simulink model "GCI_Ctrl_PLL_C2000"  (R2024a)
settings: Solver=FixedStepDiscrete  StartTime=0.0  StopTime=8  FixedStep=Sim.ContSampleTime  RelTol=1e-3  EnableMultiTasking=on
values from neighbouring files (symbols this model uses):
  ADPTV = 1.3912    [ModelDD.sldd]
  Ctrl = 0    [ModelDD.sldd]
  EnableMonitors = 0    [ModelDD.sldd]
  FrcPwr = 1    [ModelDD.sldd]
  IdSp = 0.0    [ModelDD.sldd]
  IqSp = 0.0    [ModelDD.sldd]
  ModReq = 1    [ModelDD.sldd]
  PorISel = 0    [ModelDD.sldd]
  PSp = 0.0    [ModelDD.sldd]
  QSp = 0.0    [ModelDD.sldd]
  Sim : value not decoded    [ModelDD.sldd]
  Test = 0    [ModelDD.sldd]
  Var = 650.0    [ModelDD.sldd]
undefined symbols (not defined in the file or in its folder): DiscIntNeverNeededParam, Down, GPTRIP1SEL, GPTRIP2SEL, magnitude, P, TZ1, TZ2, Up
libraries: simulink x38, c2837xDlib x22, c2802xlib x15, slpidlib x9, spsMeanLib x9, spsCurrentMeasurementLib x7, spsThreePhaseVIMeasurementLib x5, spsVoltageMeasurementLib x5, spsTHDLib x4, spsSeriesRLCBranchLib x4, svdutilitieslib x3, c280xlib x3
(part 5 of 11)

== system GCI_Ctrl_PLL_C2000/C2000_SW/CtrlLoop/PWMs/HW ==
  Duty : Inport  OutDataTypeStr=single
  SPO : Inport  Port=2
  Bias3 : Bias  Bias=-100  SaturateOnIntegerOverflow=off
  Constant : Constant  Value=single([0 0 0])
  Constant2 : Constant  Value=single(zeros(1,6))
  Demux : Demux  Outputs=3
  Gain3 : Gain  Gain=-1  ParamDataTypeStr=single
  Mux : Mux  Inputs=2
  Switch : Switch  Criteria=u2 > Threshold  SaturateOnIntegerOverflow=off  InputSameDT=off
  Switch1 : Switch  Criteria=u2 > Threshold  SaturateOnIntegerOverflow=off  InputSameDT=off
  ePWM4 : c2802xlib/ePWM  PwmType=C2000_Type4  useModule=ePWM4  ePWMxLINKTBPRD=Not Linked  periodUnits=Seconds  timerSource=Specify via dialog  timerPeriod_clk=64000  timerPeriod_sec=1/(2*Var.PWM_Freq)  tbshadow=Counter equals to zero  countingMode=Up-Down  phaseActiveEnable=Disable  phaseDirection=Count down after sync  phaseActive=0  synchronizationEnable=off  dcaevt1Sync=off  dcbevt1Sync=off  synchronizationOption=Counter equals to zero (CTR=Zero)  dcbevt1SyncOut=off  dcaevt1SyncOut=off  cmpdSyncOut=off  cmpcSyncOut=off  cmpbSyncOut=off  zeroSyncOut=on  swfSyncOut=off  perSynchronizationOption=Counter equals to period (CTR=PRD)  clockPrescale=1  HSclockPrescale=1  enswap=off  ePWMxAStatus=on  ePWMxAactionLogic1=Do nothing  ePWMxAactionLogic2=Do nothing  ePWMxAactionLogic3=Clear  ePWMxAactionLogic4=Set  ePWMxAactionLogic5=Do nothing  ePWMxAactionLogic6=Do nothing  ePWMxACSFenable=off  ePWMxACSFvalue=Forcing disable  ePWMxASFreload=Zero  ePWMxBStatus=on  ePWMxBactionLogic1=Do nothing  ePWMxBactionLogic2=Do nothing  ePWMxBactionLogic3=Set  ePWMxBactionLogic4=Clear  ePWMxBactionLogic5=Do nothing  ePWMxBactionLogic6=Do nothing  ePWMxBCSFenable=off  ePWMxBCSFvalue=Forcing disable  ePWMxBSFreload=Zero  ePWNxBOutWay=off  ePWMxLINKCMPA=Not Linked  CMPAUnits=Percentages  CMPASource=Input port  CMPAValue_per=0  CMPAValue_clk=32000  enCMPAshadow=Counter equals to period (CTR=PRD)  ePWMxLINKCMPB=Not Linked  CMPBUnits=Percentages  CMPBSource=Specify via dialog  CMPBValue_per=100  CMPBValue_clk=32000  enCMPBshadow=Counter equals to period (CTR=PRD)  ePWMxLINKCMPC=Not Linked  CMPCUnits=Clock cycles  CMPCSource=Specify via dialog  CMPCValue_per=50  CMPCValue_clk=32000  enCMPCshadow=Counter equals to zero (CTR=Zero)  ePWMxLINKCMPD=Not Linked  CMPDUnits=Clock cycles  CMPDSource=Specify via dialog  CMPDValue_per=50  CMPDValue_clk=32000  enCMPDshadow=Counter equals to zero (CTR=Zero)  enableDBePWMxA=on  enableDBePWMxB=on  enhalfcycle=off  DBpolarity=Active high complementary (AHC)  DBedgeDelay=Positive  DBSource_ePWMxA=ePWMxA  DBSource_ePWMxB=ePWMxA  DBPeriodUnits=Clock cycles  DBperiodSource=Specify via dialog  REDperiod=Var.PWM_Deadtime*1e8  FEDperiod=Var.PWM_Deadtime*1e8  REDperiod_sec=0  FEDperiod_sec=0  LoadModeDBRED=Immediate without using shadow  LoadModeDBFED=Immediate without using shadow  adcstartModuleA=on  adcrequestEventA=First event  adcstartEventA=Digital Compare Module A Event 1 start of conversion (DCAEVT1.soc)  adcstartEventA_type2=Counter equals to period (CTR=PRD)  adcstartModuleB=off  adcrequestEventB=First event  adcstartEventB=Counter equals to zero (CTR=Zero)  adcstartEventB_type2=Counter equals to period (CTR=PRD)  intEn=on  intPrd=First event  intSel=Counter equals to zero (CTR=Zero)  intSel_type2=Counter equals to period (CTR=PRD)  hrpe=off  enHRPWM=off  HRPWM_LoadMode=Counter equals to either zero or period (CTR=ZERO or CTR=PRD)  HRPWM_CTLMode=Duty or Period control mode  HRPWM_EDGMode=Both edge  hrpeb=off  enHRPWMB=off  HRPWM_LoadModeB=Counter equals to zero (CTR=ZERO)  HRPWM_CTLModeB=Duty or Period control mode  HRPWM_EDGModeB=Both edge  enHRDBRED=off  enHRDBFED=off  enSFO=on  enautoconv=on  chopperEnable=off  chopperFrequency=1  chopperFirstwidth=1  chopperDuty=12.5%  tripZonesource=Specify via dialog  tzselOSHT1=off  tzselOSHT2=off  tzselOSHT3=off  tzselOSHT4=off  tzselOSHT5=off  tzselOSHT6=off  tzselOSHDCAEV1=off  tzselOSHDCBEV1=off  tzselCBC1=on  tzselCBC2=off  tzselCBC3=off  tzselCBC4=off  tzselCBC5=off  tzselCBC6=off  tzselCBCDCAEV2=off  tzselCBCDCBEV2=off  enTzOstIntr=off  enTzCbcIntr=off  enTzDCAEVT1Intr=off  enTzDCAEVT2Intr=off  enTzDCBEVT1Intr=off  enTzDCBEVT2Intr=off  tzclrCBCLatch=Counter equals to zero (CTR=Zero)  ePWMxAforced=Low  ePWMxBforced=Low  DCAEVT1forced=No action  DCBEVT1forced=No action  DCAEVT2forced=No action  DCBEVT2forced=No action  dcah=Trip Zone 1 input (TZ1)  dcal=Trip Zone 2 input (TZ2)  dcbh=Trip Zone 1 input (TZ1)  dcbl=Trip Zone 2 input (TZ2)  dcah_type2=GPTRIP1SEL/(TZ1)  dcal_type2=GPTRIP2SEL/(TZ2)  dcbh_type2=GPTRIP1SEL/(TZ1)  dcbl_type2=GPTRIP2SEL/(TZ2)  gendcaevt1=Event disabled  gendcaevt2=Event disabled  gendcbevt1=Event disabled  gendcbevt2=Event disabled  dcaevt1src=DCAEVT1 with sync  dcaevt2src=DCAEVT2 with sync  dcbevt1src=DCBEVT1 with sync  dcbevt2src=DCBEVT2 with sync  pulsesel=Counter equals to zero (CTR=Zero)  blankinv=off  blankoffset=0  blankwidth=0  evsrcsel=Filtered version of DCAEVT1 (DCAEVT1FILT)  encape=off
  ePWM5 : c2802xlib/ePWM  PwmType=C2000_Type4  useModule=ePWM5  ePWMxLINKTBPRD=Not Linked  periodUnits=Seconds  timerSource=Specify via dialog  timerPeriod_clk=64000  timerPeriod_sec=1/(2*Var.PWM_Freq)  tbshadow=Counter equals to zero  countingMode=Up-Down  phaseActiveEnable=Set counter to phase value specified via dialog  phaseDirection=Count up after sync  phaseActive=0  synchronizationEnable=off  dcaevt1Sync=off  dcbevt1Sync=off  synchronizationOption=Pass through (EPWMxSYNCI or SWFSYNC)  dcbevt1SyncOut=off  dcaevt1SyncOut=off  cmpdSyncOut=off  cmpcSyncOut=off  cmpbSyncOut=off  zeroSyncOut=off  swfSyncOut=on  perSynchronizationOption=Counter equals to period (CTR=PRD)  clockPrescale=1  HSclockPrescale=1  enswap=off  ePWMxAStatus=on  ePWMxAactionLogic1=Do nothing  ePWMxAactionLogic2=Do nothing  ePWMxAactionLogic3=Clear  ePWMxAactionLogic4=Set  ePWMxAactionLogic5=Do nothing  ePWMxAactionLogic6=Do nothing  ePWMxACSFenable=off  ePWMxACSFvalue=Forcing disable  ePWMxASFreload=Zero  ePWMxBStatus=on  ePWMxBactionLogic1=Do nothing  ePWMxBactionLogic2=Do nothing  ePWMxBactionLogic3=Set  ePWMxBactionLogic4=Clear  ePWMxBactionLogic5=Do nothing  ePWMxBactionLogic6=Do nothing  ePWMxBCSFenable=off  ePWMxBCSFvalue=Forcing disable  ePWMxBSFreload=Zero  ePWNxBOutWay=off  ePWMxLINKCMPA=Not Linked  CMPAUnits=Percentages  CMPASource=Input port  CMPAValue_per=0  CMPAValue_clk=32000  enCMPAshadow=Counter equals to period (CTR=PRD)  ePWMxLINKCMPB=Not Linked  CMPBUnits=Percentages  CMPBSource=Specify via dialog  CMPBValue_per=100  CMPBValue_clk=32000  enCMPBshadow=Counter equals to period (CTR=PRD)  ePWMxLINKCMPC=Not Linked  CMPCUnits=Clock cycles  CMPCSource=Specify via dialog  CMPCValue_per=50  CMPCValue_clk=32000  enCMPCshadow=Counter equals to zero (CTR=Zero)  ePWMxLINKCMPD=Not Linked  CMPDUnits=Clock cycles  CMPDSource=Specify via dialog  CMPDValue_per=50  CMPDValue_clk=32000  enCMPDshadow=Counter equals to zero (CTR=Zero)  enableDBePWMxA=on  enableDBePWMxB=on  enhalfcycle=off  DBpolarity=Active high complementary (AHC)  DBedgeDelay=Positive  DBSource_ePWMxA=ePWMxA  DBSource_ePWMxB=ePWMxA  DBPeriodUnits=Clock cycles  DBperiodSource=Specify via dialog  REDperiod=Var.PWM_Deadtime*1e8  FEDperiod=Var.PWM_Deadtime*1e8  REDperiod_sec=0  FEDperiod_sec=0  LoadModeDBRED=Immediate without using shadow  LoadModeDBFED=Immediate without using shadow  adcstartModuleA=off  adcrequestEventA=First event  adcstartEventA=Digital Compare Module A Event 1 start of conversion (DCAEVT1.soc)  adcstartEventA_type2=Digital Compare Module A Event 1 start of conversion (DCAEVT1.soc)  adcstartModuleB=off  adcrequestEventB=First event  adcstartEventB=Counter equals to zero (CTR=Zero)  adcstartEventB_type2=Counter equals to zero (CTR=Zero)  intEn=off  intPrd=First event  intSel=Counter equals to zero (CTR=Zero)  intSel_type2=Counter equals to zero (CTR=Zero)  hrpe=off  enHRPWM=off  HRPWM_LoadMode=Counter equals to either zero or period (CTR=ZERO or CTR=PRD)  HRPWM_CTLMode=Duty or Period control mode  HRPWM_EDGMode=Both edge  hrpeb=off  enHRPWMB=off  HRPWM_LoadModeB=Counter equals to zero (CTR=ZERO)  HRPWM_CTLModeB=Duty or Period control mode  HRPWM_EDGModeB=Both edge  enHRDBRED=off  enHRDBFED=off  enSFO=on  enautoconv=on  chopperEnable=off  chopperFrequency=1  chopperFirstwidth=1  chopperDuty=12.5%  tripZonesource=Specify via dialog  tzselOSHT1=off  tzselOSHT2=off  tzselOSHT3=off  tzselOSHT4=off  tzselOSHT5=off  tzselOSHT6=off  tzselOSHDCAEV1=off  tzselOSHDCBEV1=off  tzselCBC1=on  tzselCBC2=off  tzselCBC3=off  tzselCBC4=off  tzselCBC5=off  tzselCBC6=off  tzselCBCDCAEV2=off  tzselCBCDCBEV2=off  enTzOstIntr=off  enTzCbcIntr=off  enTzDCAEVT1Intr=off  enTzDCAEVT2Intr=off  enTzDCBEVT1Intr=off  enTzDCBEVT2Intr=off  tzclrCBCLatch=Counter equals to zero (CTR=Zero)  ePWMxAforced=Low  ePWMxBforced=Low  DCAEVT1forced=No action  DCBEVT1forced=No action  DCAEVT2forced=No action  DCBEVT2forced=No action  dcah=Trip Zone 1 input (TZ1)  dcal=Trip Zone 2 input (TZ2)  dcbh=Trip Zone 1 input (TZ1)  dcbl=Trip Zone 2 input (TZ2)  dcah_type2=GPTRIP1SEL/(TZ1)  dcal_type2=GPTRIP2SEL/(TZ2)  dcbh_type2=GPTRIP1SEL/(TZ1)  dcbl_type2=GPTRIP2SEL/(TZ2)  gendcaevt1=Event disabled  gendcaevt2=Event disabled  gendcbevt1=Event disabled  gendcbevt2=Event disabled  dcaevt1src=DCAEVT1 with sync  dcaevt2src=DCAEVT2 with sync  dcbevt1src=DCBEVT1 with sync  dcbevt2src=DCBEVT2 with sync  pulsesel=Counter equals to zero (CTR=Zero)  blankinv=off  blankoffset=0  blankwidth=0  evsrcsel=Filtered version of DCAEVT1 (DCAEVT1FILT)  encape=off
  ePWM6 : c2802xlib/ePWM  PwmType=C2000_Type4  useModule=ePWM6  ePWMxLINKTBPRD=Not Linked  periodUnits=Seconds  timerSource=Specify via dialog  timerPeriod_clk=64000  timerPeriod_sec=1/(2*Var.PWM_Freq)  tbshadow=Counter equals to zero  countingMode=Up-Down  phaseActiveEnable=Set counter to phase value specified via dialog  phaseDirection=Count up after sync  phaseActive=0  synchronizationEnable=off  dcaevt1Sync=off  dcbevt1Sync=off  synchronizationOption=Disable  dcbevt1SyncOut=off  dcaevt1SyncOut=off  cmpdSyncOut=off  cmpcSyncOut=off  cmpbSyncOut=off  zeroSyncOut=off  swfSyncOut=off  perSynchronizationOption=Counter equals to period (CTR=PRD)  clockPrescale=1  HSclockPrescale=1  enswap=off  ePWMxAStatus=on  ePWMxAactionLogic1=Do nothing  ePWMxAactionLogic2=Do nothing  ePWMxAactionLogic3=Clear  ePWMxAactionLogic4=Set  ePWMxAactionLogic5=Do nothing  ePWMxAactionLogic6=Do nothing  ePWMxACSFenable=off  ePWMxACSFvalue=Forcing disable  ePWMxASFreload=Zero  ePWMxBStatus=on  ePWMxBactionLogic1=Do nothing  ePWMxBactionLogic2=Do nothing  ePWMxBactionLogic3=Set  ePWMxBactionLogic4=Clear  ePWMxBactionLogic5=Do nothing  ePWMxBactionLogic6=Do nothing  ePWMxBCSFenable=off  ePWMxBCSFvalue=Forcing disable  ePWMxBSFreload=Zero  ePWNxBOutWay=off  ePWMxLINKCMPA=Not Linked  CMPAUnits=Percentages  CMPASource=Input port  CMPAValue_per=0  CMPAValue_clk=32000  enCMPAshadow=Counter equals to period (CTR=PRD)  ePWMxLINKCMPB=Not Linked  CMPBUnits=Percentages  CMPBSource=Specify via dialog  CMPBValue_per=100  CMPBValue_clk=32000  enCMPBshadow=Counter equals to period (CTR=PRD)  ePWMxLINKCMPC=Not Linked  CMPCUnits=Clock cycles  CMPCSource=Specify via dialog  CMPCValue_per=50  CMPCValue_clk=32000  enCMPCshadow=Counter equals to zero (CTR=Zero)  ePWMxLINKCMPD=Not Linked  CMPDUnits=Clock cycles  CMPDSource=Specify via dialog  CMPDValue_per=50  CMPDValue_clk=32000  enCMPDshadow=Counter equals to zero (CTR=Zero)  enableDBePWMxA=on  enableDBePWMxB=on  enhalfcycle=off  DBpolarity=Active high complementary (AHC)  DBedgeDelay=Positive  DBSource_ePWMxA=ePWMxA  DBSource_ePWMxB=ePWMxA  DBPeriodUnits=Clock cycles  DBperiodSource=Specify via dialog  REDperiod=Var.PWM_Deadtime*1e8  FEDperiod=Var.PWM_Deadtime*1e8  REDperiod_sec=0  FEDperiod_sec=0  LoadModeDBRED=Immediate without using shadow  LoadModeDBFED=Immediate without using shadow  adcstartModuleA=off  adcrequestEventA=First event  adcstartEventA=Digital Compare Module A Event 1 start of conversion (DCAEVT1.soc)  adcstartEventA_type2=Digital Compare Module A Event 1 start of conversion (DCAEVT1.soc)  adcstartModuleB=off  adcrequestEventB=First event  adcstartEventB=Counter equals to zero (CTR=Zero)  adcstartEventB_type2=Counter equals to zero (CTR=Zero)  intEn=off  intPrd=First event  intSel=Counter equals to zero (CTR=Zero)  intSel_type2=Counter equals to zero (CTR=Zero)  hrpe=off  enHRPWM=off  HRPWM_LoadMode=Counter equals to either zero or period (CTR=ZERO or CTR=PRD)  HRPWM_CTLMode=Duty or Period control mode  HRPWM_EDGMode=Both edge  hrpeb=off  enHRPWMB=off  HRPWM_LoadModeB=Counter equals to zero (CTR=ZERO)  HRPWM_CTLModeB=Duty or Period control mode  HRPWM_EDGModeB=Both edge  enHRDBRED=off  enHRDBFED=off  enSFO=on  enautoconv=on  chopperEnable=off  chopperFrequency=1  chopperFirstwidth=1  chopperDuty=12.5%  tripZonesource=Specify via dialog  tzselOSHT1=off  tzselOSHT2=off  tzselOSHT3=off  tzselOSHT4=off  tzselOSHT5=off  tzselOSHT6=off  tzselOSHDCAEV1=off  tzselOSHDCBEV1=off  tzselCBC1=on  tzselCBC2=off  tzselCBC3=off  tzselCBC4=off  tzselCBC5=off  tzselCBC6=off  tzselCBCDCAEV2=off  tzselCBCDCBEV2=off  enTzOstIntr=off  enTzCbcIntr=off  enTzDCAEVT1Intr=off  enTzDCAEVT2Intr=off  enTzDCBEVT1Intr=off  enTzDCBEVT2Intr=off  tzclrCBCLatch=Counter equals to zero (CTR=Zero)  ePWMxAforced=Low  ePWMxBforced=Low  DCAEVT1forced=No action  DCBEVT1forced=No action  DCAEVT2forced=No action  DCBEVT2forced=No action  dcah=Trip Zone 1 input (TZ1)  dcal=Trip Zone 2 input (TZ2)  dcbh=Trip Zone 1 input (TZ1)  dcbl=Trip Zone 2 input (TZ2)  dcah_type2=GPTRIP1SEL/(TZ1)  dcal_type2=GPTRIP2SEL/(TZ2)  dcbh_type2=GPTRIP1SEL/(TZ1)  dcbl_type2=GPTRIP2SEL/(TZ2)  gendcaevt1=Event disabled  gendcaevt2=Event disabled  gendcbevt1=Event disabled  gendcbevt2=Event disabled  dcaevt1src=DCAEVT1 with sync  dcaevt2src=DCAEVT2 with sync  dcbevt1src=DCBEVT1 with sync  dcbevt2src=DCBEVT2 with sync  pulsesel=Counter equals to zero (CTR=Zero)  blankinv=off  blankoffset=0  blankwidth=0  evsrcsel=Filtered version of DCAEVT1 (DCAEVT1FILT)  encape=off
  DutyOut : Outport  VectorParamsAs1DForOutWhenUnconnected=off
  wires:
  Switch/1 -> Demux/1, Mux/1, Bias3/1
  Demux/1 -> ePWM4/1
  Switch1/1 -> DutyOut/1
  Demux/3 -> ePWM6/1
  Duty/1 -> Switch/3
  Constant/1 -> Switch/1
  Demux/2 -> ePWM5/1
  Constant2/1 -> Switch1/1
  SPO/1 -> [A1]
  [A1] -> Switch1/2
  [A1] -> Switch/2
  Bias3/1 -> Gain3/1
  Gain3/1 -> Mux/2
  Mux/1 -> Switch1/3

== system GCI_Ctrl_PLL_C2000/C2000_SW/CtrlLoop/PWMs/SIM ==
  Duty : Inport  OutDataTypeStr=single
  SPO : Inport  Port=2
  Bias2 : Bias  Bias=-100  SaturateOnIntegerOverflow=off
  Constant : Constant  OutDataTypeStr=boolean
  Constant1 : Constant  Value=single([0 0 0 0 0 0])
  Gain1 : Gain  Gain=-1  ParamDataTypeStr=single
  Manual Switch : ManualSwitch  CurrentSetting=0
  Mux : Mux  Inputs=2
  Switch : Switch  Criteria=u2 > Threshold  SaturateOnIntegerOverflow=off  InputSameDT=off
  DutyOut : Outport  VectorParamsAs1DForOutWhenUnconnected=off
  wires:
  Manual Switch/1 -> Switch/2
  Duty/1 -> Mux/1, Bias2/1
  Constant/1 -> Manual Switch/1
  Constant1/1 -> Switch/1
  Switch/1 -> DutyOut/1  "DutyOut"
  Mux/1 -> Switch/3
  SPO/1 -> Manual Switch/2
  Bias2/1 -> Gain1/1
  Gain1/1 -> Mux/2

== system GCI_Ctrl_PLL_C2000/C2000_SW/CtrlLoop/RMS/LPF2 ==
  u : Inport
  Alpha : Gain  Gain=(2-w*Ts)/(2+w*Ts)
  Beta : Gain  Gain=(w*Ts)/(2+w*Ts)
  Delay1 : Delay  DelayLength=1  InitialCondition=y_0
  Delay2 : Delay  DelayLength=1
  Sum1 : Sum  Inputs=++|
  Sum2 : Sum  Inputs=|++
  y : Outport  VectorParamsAs1DForOutWhenUnconnected=off
  wires:
  Sum2/1 -> y/1, Delay1/1
  Beta/1 -> Sum2/1
  Sum1/1 -> Beta/1
  Delay2/1 -> Sum1/2
  Alpha/1 -> Sum2/2
  Delay1/1 -> Alpha/1  "y(n-1)"
  u/1 -> Delay2/1, Sum1/1

== system GCI_Ctrl_PLL_C2000/C2000_SW/CtrlLoop/RMS1/LPF2 ==
  u : Inport
  Alpha : Gain  Gain=(2-w*Ts)/(2+w*Ts)
  Beta : Gain  Gain=(w*Ts)/(2+w*Ts)
  Delay1 : Delay  DelayLength=1  InitialCondition=y_0
  Delay2 : Delay  DelayLength=1
  Sum1 : Sum  Inputs=++|
  Sum2 : Sum  Inputs=|++
  y : Outport  VectorParamsAs1DForOutWhenUnconnected=off
  wires:
  u/1 -> Sum1/1, Delay2/1
  Delay1/1 -> Alpha/1  "y(n-1)"
  Alpha/1 -> Sum2/2
  Delay2/1 -> Sum1/2
  Sum1/1 -> Beta/1
  Beta/1 -> Sum2/1
  Sum2/1 -> Delay1/1, y/1

== system GCI_Ctrl_PLL_C2000/C2000_SW/MnrErr/Monitoring/ADC_OORH ==
  u : Inport
  Bias : Bias  Bias=single(-0.5)  SaturateOnIntegerOverflow=off
  Compare To Constant : simulink/Logic and Bit Operations/Compare To Constant  relop=>=  const=Lim  OutDataTypeStr=uint8
  Compare To Constant1 : simulink/Logic and Bit Operations/Compare To Constant  relop===  const=single(2)  OutDataTypeStr=boolean
  Compare To Constant2 : simulink/Logic and Bit Operations/Compare To Constant  relop===  const=single(-1.5)  OutDataTypeStr=boolean
  Compare To Constant3 : simulink/Logic and Bit Operations/Compare To Constant  relop=<=  const=LimN  OutDataTypeStr=uint8
  Constant : Constant  Value=single(0)
  Constant1 : Constant  Value=UorL
  Discrete-Time Integrator2 : DiscreteIntegrator  gainval=single(1/Tmon)  SampleTime=-1  OutDataTypeStr=single  LimitOutput=on  UpperSaturationLimit=single(1)  LowerSaturationLimit=single(0)  ShowSaturationPort=on  ICPrevOutput=DiscIntNeverNeededParam  ICPrevScaledInput=DiscIntNeverNeededParam
  Gain : Gain  Gain=single(1.5)  ParamDataTypeStr=single
  OR : Logic  Operator=OR  IconShape=distinctive  AllPortsSameDT=off  OutDataTypeStr=boolean
  Relay : Relay  OnSwitchValue=1  OffSwitchValue=0
  Sum : Sum  Inputs=|++
  Switch : Switch  Threshold=1  SaturateOnIntegerOverflow=off  InputSameDT=off
  Switch1 : Switch  Threshold=1  SaturateOnIntegerOverflow=off  InputSameDT=off
  Unit Delay : UnitDelay  SampleTime=-1  HasFrameUpgradeWarning=on
  err : Outport
  wires:
  Unit Delay/1 -> Sum/1
  Discrete-Time Integrator2/1 -> Relay/1
  Constant/1 -> Switch/1
  Switch/1 -> Discrete-Time Integrator2/1
  Discrete-Time Integrator2/2 -> Unit Delay/1
  Relay/1 -> err/1
  Sum/1 -> Compare To Constant2/1, Compare To Constant1/1
  Compare To Constant2/1 -> OR/1
  Compare To Constant1/1 -> OR/2
  OR/1 -> Switch/2
  Switch1/1 -> Gain/1
  Gain/1 -> Bias/1
  Bias/1 -> Switch/3, Sum/2
  Compare To Constant3/1 -> Switch1/3
  Compare To Constant/1 -> Switch1/1
  Constant1/1 -> Switch1/2
  u/1 -> Compare To Constant/1, Compare To Constant3/1

== system GCI_Ctrl_PLL_C2000/C2000_SW/MnrErr/Monitoring/ADC_OORL ==
  u : Inport
  Bias : Bias  Bias=single(-0.5)  SaturateOnIntegerOverflow=off
  Compare To Constant : simulink/Logic and Bit Operations/Compare To Constant  relop=>=  const=Lim  OutDataTypeStr=uint8
  Compare To Constant1 : simulink/Logic and Bit Operations/Compare To Constant  relop===  const=single(2)  OutDataTypeStr=boolean
  Compare To Constant2 : simulink/Logic and Bit Operations/Compare To Constant  relop===  const=single(-1.5)  OutDataTypeStr=boolean
  Compare To Constant3 : simulink/Logic and Bit Operations/Compare To Constant  relop=<=  const=LimN  OutDataTypeStr=uint8
  Constant : Constant  Value=single(0)
  Constant1 : Constant  Value=UorL
  Discrete-Time Integrator2 : DiscreteIntegrator  gainval=single(1/Tmon)  SampleTime=-1  OutDataTypeStr=single  LimitOutput=on  UpperSaturationLimit=single(1)  LowerSaturationLimit=single(0)  ShowSaturationPort=on  ICPrevOutput=DiscIntNeverNeededParam  ICPrevScaledInput=DiscIntNeverNeededParam
  Gain : Gain  Gain=single(1.5)  ParamDataTypeStr=single
  OR : Logic  Operator=OR  IconShape=distinctive  AllPortsSameDT=off  OutDataTypeStr=boolean
  Relay : Relay  OnSwitchValue=1  OffSwitchValue=0
  Sum : Sum  Inputs=|++
  Switch : Switch  Threshold=1  SaturateOnIntegerOverflow=off  InputSameDT=off
  Switch1 : Switch  Threshold=1  SaturateOnIntegerOverflow=off  InputSameDT=off
  Unit Delay : UnitDelay  SampleTime=-1  HasFrameUpgradeWarning=on
  err : Outport
  wires:
  u/1 -> Compare To Constant3/1, Compare To Constant/1
  Constant1/1 -> Switch1/2
  Compare To Constant/1 -> Switch1/1
  Compare To Constant3/1 -> Switch1/3
  Bias/1 -> Sum/2, Switch/3
  Gain/1 -> Bias/1
  Switch1/1 -> Gain/1
  OR/1 -> Switch/2
  Compare To Constant1/1 -> OR/2
  Compare To Constant2/1 -> OR/1
  Sum/1 -> Compare To Constant1/1, Compare To Constant2/1
  Relay/1 -> err/1
  Discrete-Time Integrator2/2 -> Unit Delay/1
  Switch/1 -> Discrete-Time Integrator2/1
  Constant/1 -> Switch/1
  Discrete-Time Integrator2/1 -> Relay/1
  Unit Delay/1 -> Sum/1

== system GCI_Ctrl_PLL_C2000/C2000_SW/MnrErr/Monitoring/HvdcUOV ==
  u : Inport
  Bias : Bias  Bias=single(-0.01)  SaturateOnIntegerOverflow=off
  Compare To Constant : simulink/Logic and Bit Operations/Compare To Constant  relop=>=  const=Lim  OutDataTypeStr=uint8
  Compare To Constant1 : simulink/Logic and Bit Operations/Compare To Constant  relop===  const=single(2)  OutDataTypeStr=boolean
  Compare To Constant2 : simulink/Logic and Bit Operations/Compare To Constant  relop===  const=single(-1.5)  OutDataTypeStr=boolean
  Compare To Constant3 : simulink/Logic and Bit Operations/Compare To Constant  relop=<=  const=LimN  OutDataTypeStr=uint8
  Constant : Constant  Value=single(0)
  Constant1 : Constant  Value=UorL
  Discrete-Time Integrator2 : DiscreteIntegrator  gainval=single(1/Tmon)  SampleTime=-1  OutDataTypeStr=single  LimitOutput=on  UpperSaturationLimit=single(1)  LowerSaturationLimit=single(0)  ShowSaturationPort=on  ICPrevOutput=DiscIntNeverNeededParam  ICPrevScaledInput=DiscIntNeverNeededParam
  Gain : Gain  Gain=single(1.01)  ParamDataTypeStr=single
  OR : Logic  Operator=OR  IconShape=distinctive  AllPortsSameDT=off  OutDataTypeStr=boolean
  Relay : Relay  OnSwitchValue=1  OffSwitchValue=0
  Sum : Sum  Inputs=|++
  Switch : Switch  Threshold=1  SaturateOnIntegerOverflow=off  InputSameDT=off
  Switch1 : Switch  Threshold=1  SaturateOnIntegerOverflow=off  InputSameDT=off
  Unit Delay : UnitDelay  SampleTime=-1  HasFrameUpgradeWarning=on
  err : Outport
  wires:
  u/1 -> Compare To Constant3/1, Compare To Constant/1
  Constant1/1 -> Switch1/2
  Compare To Constant/1 -> Switch1/1
  Compare To Constant3/1 -> Switch1/3
  Bias/1 -> Sum/2, Switch/3
  Gain/1 -> Bias/1
  Switch1/1 -> Gain/1
  OR/1 -> Switch/2
  Compare To Constant1/1 -> OR/2
  Compare To Constant2/1 -> OR/1
  Sum/1 -> Compare To Constant1/1, Compare To Constant2/1
  Relay/1 -> err/1
  Discrete-Time Integrator2/2 -> Unit Delay/1
  Switch/1 -> Discrete-Time Integrator2/1
  Constant/1 -> Switch/1
  Discrete-Time Integrator2/1 -> Relay/1
  Unit Delay/1 -> Sum/1

== system GCI_Ctrl_PLL_C2000/C2000_SW/MnrErr/Monitoring/RMS_OC ==
  u : Inport
  Bias : Bias  Bias=single(-0.01)  SaturateOnIntegerOverflow=off
  Compare To Constant : simulink/Logic and Bit Operations/Compare To Constant  relop=>=  const=Lim  OutDataTypeStr=uint8
  Compare To Constant1 : simulink/Logic and Bit Operations/Compare To Constant  relop===  const=single(2)  OutDataTypeStr=boolean
  Compare To Constant2 : simulink/Logic and Bit Operations/Compare To Constant  relop===  const=single(-1.5)  OutDataTypeStr=boolean
  Compare To Constant3 : simulink/Logic and Bit Operations/Compare To Constant  relop=<=  const=LimN  OutDataTypeStr=uint8
  Constant : Constant  Value=single(0)
  Constant1 : Constant  Value=UorL
  Discrete-Time Integrator2 : DiscreteIntegrator  gainval=single(1/Tmon)  SampleTime=-1  OutDataTypeStr=single  LimitOutput=on  UpperSaturationLimit=single(1)  LowerSaturationLimit=single(0)  ShowSaturationPort=on  ICPrevOutput=DiscIntNeverNeededParam  ICPrevScaledInput=DiscIntNeverNeededParam
  Gain : Gain  Gain=single(1.01)  ParamDataTypeStr=single
  OR : Logic  Operator=OR  IconShape=distinctive  AllPortsSameDT=off  OutDataTypeStr=boolean
  Relay : Relay  OnSwitchValue=1  OffSwitchValue=0
  Sum : Sum  Inputs=|++
  Switch : Switch  Threshold=1  SaturateOnIntegerOverflow=off  InputSameDT=off
  Switch1 : Switch  Threshold=1  SaturateOnIntegerOverflow=off  InputSameDT=off
  Unit Delay : UnitDelay  SampleTime=-1  HasFrameUpgradeWarning=on
  err : Outport
  wires:
  Unit Delay/1 -> Sum/1
  Discrete-Time Integrator2/1 -> Relay/1
  Constant/1 -> Switch/1
  Switch/1 -> Discrete-Time Integrator2/1
  Discrete-Time Integrator2/2 -> Unit Delay/1
  Relay/1 -> err/1
  Sum/1 -> Compare To Constant2/1, Compare To Constant1/1
  Compare To Constant2/1 -> OR/1
  Compare To Constant1/1 -> OR/2
  OR/1 -> Switch/2
  Switch1/1 -> Gain/1
  Gain/1 -> Bias/1
  Bias/1 -> Switch/3, Sum/2
  Compare To Constant3/1 -> Switch1/3
  Compare To Constant/1 -> Switch1/1
  Constant1/1 -> Switch1/2
  u/1 -> Compare To Constant/1, Compare To Constant3/1

== system GCI_Ctrl_PLL_C2000/PowerSystem/Actual System/PWMGen2/Deadtime ==
  In1 : Inport
  AND : Logic  IconShape=distinctive  AllPortsSameDT=off  OutDataTypeStr=boolean
  Data Type Conversion : DataTypeConversion  OutDataTypeStr=double  SaturateOnIntegerOverflow=off  RndMeth=Floor
  Data Type Conversion1 : DataTypeConversion  SaturateOnIntegerOverflow=off  RndMeth=Floor
  Transport Delay : TransportDelay  DelayTime=double(Var.PWM.Freq)
  Out1 : Outport  VectorParamsAs1DForOutWhenUnconnected=off
  wires:
  Transport Delay/1 -> AND/1
  In1/1 -> Data Type Conversion/1
  AND/1 -> Data Type Conversion1/1
  Data Type Conversion/1 -> Transport Delay/1, AND/2
  Data Type Conversion1/1 -> Out1/1

== system GCI_Ctrl_PLL_C2000/PowerSystem/Meas/Fault Injection/3PhaseToGnd ==
  Add7 : Sum
  Constant : Constant  Value=Mag
  Constant1 : Constant  Value=Frq*2*pi
  Constant2 : Constant  Value=Pha*pi/180
  Constant3 : Constant  Value=HarmOrd  VectorParams1D=off
  Constant4 : Constant  Value=IntHarmOrd  VectorParams1D=off
  Constant5 : Constant  Value=2*pi
  Cos1 : Trigonometry  Operator=cos
  Cos3 : Trigonometry  Operator=cos
  Cos8 : Trigonometry  Operator=cos
  Discrete-Time Integrator2 : DiscreteIntegrator  IntegratorMethod=Integration: Trapezoidal  SampleTime=-1  ICPrevOutput=DiscIntNeverNeededParam  ICPrevScaledInput=DiscIntNeverNeededParam
  Frq : Step  Time=FrqStpT  After=FrqStp*2*pi  SampleTime=0
  Gain : Gain  Gain=DcOff
  Harm : Step  Time=HarmStp  After=Harm  SampleTime=0  VectorParams1D=off
  Harm1 : Step  Time=IntHarmStp  After=IntHarm  SampleTime=0  VectorParams1D=off
  Mag : Step  Time=MagStpT  Before=1  After=MagStpPerc  SampleTime=0
  Matrix Multiply{,1..3} (4 alike) : Product  Multiplication=Matrix(*)
  Mod : Math  Operator=mod  SignedPower=on
  Phase : Step  Time=PhaStpT  After=(PhaStpPerc)*pi/180  SampleTime=0
  Product{,1,3,8} (4 alike) : Product
  Sum : Sum  Inputs=|++
  Sum of Elements : Sum  Inputs=+  CollapseMode=Specified dimension  CollapseDim=2
  Sum of Elements1 : Sum  Inputs=+  CollapseMode=Specified dimension  CollapseDim=2
  Sum of Elements2 : Sum  Inputs=+
  Sum1 : Sum  Inputs=|++
  Sum2 : Sum  Inputs=+--
  Sum3 : Sum  Inputs=++|
  Uact : Scope  NumInputPorts=2
  Wave : Outport  VectorParamsAs1DForOutWhenUnconnected=off
  wires:
  Sum of Elements2/1 -> Sum/2
  Mod/1 -> Uact/1  "wt_act"
  Constant5/1 -> Mod/2
  Gain/1 -> Sum3/1
  Sum3/1 -> Wave/1, Uact/2  "Uabc_act"
  Add7/1 -> Matrix Multiply/1, Matrix Multiply2/1, Cos3/1
  Product/1 -> Gain/1, Product3/2, Matrix Multiply1/1, Matrix Multiply3/1
  Matrix Multiply2/1 -> Cos1/1
  Matrix Multiply3/1 -> Product1/1
  Cos1/1 -> Product1/2
  Product1/1 -> Sum of Elements1/1
  Constant4/1 -> Matrix Multiply2/2
  Harm1/1 -> Matrix Multiply3/2
  Sum of Elements1/1 -> Sum2/3
  Sum2/1 -> Sum3/2
  Sum of Elements/1 -> Sum2/2
  Harm/1 -> Matrix Multiply1/2
  Constant3/1 -> Matrix Multiply/2
  Product8/1 -> Sum of Elements/1
  Cos8/1 -> Product8/2
  Matrix Multiply1/1 -> Product8/1
  Matrix Multiply/1 -> Cos8/1
  Constant2/1 -> Sum1/1
  Phase/1 -> Sum1/2
  Constant/1 -> Product/1
  Mag/1 -> Product/2
  Frq/1 -> Sum of Elements2/1
  Constant1/1 -> Sum/1
  Sum/1 -> Discrete-Time Integrator2/1
  Discrete-Time Integrator2/1 -> Add7/1, Mod/1  "wt_act"
  Product3/1 -> Sum2/1
  Sum1/1 -> Add7/2
  Cos3/1 -> Product3/1

== system GCI_Ctrl_PLL_C2000/PowerSystem/Meas/Fault Injection/FreqVar ==
  Add7 : Sum
  Constant : Constant  Value=Mag
  Constant1 : Constant  Value=Frq*2*pi
  Constant2 : Constant  Value=Pha*pi/180
  Constant3 : Constant  Value=HarmOrd  VectorParams1D=off
  Constant4 : Constant  Value=IntHarmOrd  VectorParams1D=off
  Constant5 : Constant  Value=2*pi
  Cos1 : Trigonometry  Operator=cos
  Cos3 : Trigonometry  Operator=cos
  Cos8 : Trigonometry  Operator=cos
  Discrete-Time Integrator2 : DiscreteIntegrator  IntegratorMethod=Integration: Trapezoidal  SampleTime=-1  ICPrevOutput=DiscIntNeverNeededParam  ICPrevScaledInput=DiscIntNeverNeededParam
  Frq : Step  Time=FrqStpT  After=FrqStp*2*pi  SampleTime=0
  Gain : Gain  Gain=DcOff
  Harm : Step  Time=HarmStp  After=Harm  SampleTime=0  VectorParams1D=off
  Harm1 : Step  Time=IntHarmStp  After=IntHarm  SampleTime=0  VectorParams1D=off
  Mag : Step  Time=MagStpT  Before=1  After=MagStpPerc  SampleTime=0
  Matrix Multiply{,1..3} (4 alike) : Product  Multiplication=Matrix(*)
  Mod : Math  Operator=mod  SignedPower=on
  Phase : Step  Time=PhaStpT  After=(PhaStpPerc)*pi/180  SampleTime=0
  Product{,1,3,8} (4 alike) : Product
  Sum : Sum  Inputs=|++
  Sum of Elements : Sum  Inputs=+  CollapseMode=Specified dimension  CollapseDim=2
  Sum of Elements1 : Sum  Inputs=+  CollapseMode=Specified dimension  CollapseDim=2
  Sum of Elements2 : Sum  Inputs=+
  Sum1 : Sum  Inputs=|++
  Sum2 : Sum  Inputs=+--
  Sum3 : Sum  Inputs=++|
  Uact : Scope  NumInputPorts=2
  Wave : Outport  VectorParamsAs1DForOutWhenUnconnected=off
  wires:
  Cos3/1 -> Product3/1
  Sum1/1 -> Add7/2
  Product3/1 -> Sum2/1
  Discrete-Time Integrator2/1 -> Mod/1, Add7/1  "wt_act"
  Sum/1 -> Discrete-Time Integrator2/1
  Constant1/1 -> Sum/1
  Frq/1 -> Sum of Elements2/1
  Mag/1 -> Product/2
  Constant/1 -> Product/1
  Phase/1 -> Sum1/2
  Constant2/1 -> Sum1/1
  Matrix Multiply/1 -> Cos8/1
  Matrix Multiply1/1 -> Product8/1
  Cos8/1 -> Product8/2
  Product8/1 -> Sum of Elements/1
  Constant3/1 -> Matrix Multiply/2
  Harm/1 -> Matrix Multiply1/2
  Sum of Elements/1 -> Sum2/2
  Sum2/1 -> Sum3/2
  Sum of Elements1/1 -> Sum2/3
  Harm1/1 -> Matrix Multiply3/2
  Constant4/1 -> Matrix Multiply2/2
  Product1/1 -> Sum of Elements1/1
  Cos1/1 -> Product1/2
  Matrix Multiply3/1 -> Product1/1
  Matrix Multiply2/1 -> Cos1/1
  Product/1 -> Matrix Multiply3/1, Matrix Multiply1/1, Product3/2, Gain/1
  Add7/1 -> Cos3/1, Matrix Multiply2/1, Matrix Multiply/1
  Sum3/1 -> Uact/2, Wave/1  "Uabc_act"
  Gain/1 -> Sum3/1
  Constant5/1 -> Mod/2
  Mod/1 -> Uact/1  "wt_act"
  Sum of Elements2/1 -> Sum/2

== system GCI_Ctrl_PLL_C2000/PowerSystem/Meas/Fault Injection/Harm ==
  Add7 : Sum
  Constant : Constant  Value=Mag
  Constant1 : Constant  Value=Frq*2*pi
  Constant2 : Constant  Value=Pha*pi/180
  Constant3 : Constant  Value=HarmOrd  VectorParams1D=off
  Constant4 : Constant  Value=IntHarmOrd  VectorParams1D=off
  Constant5 : Constant  Value=2*pi
  Cos1 : Trigonometry  Operator=cos
  Cos3 : Trigonometry  Operator=cos
  Cos8 : Trigonometry  Operator=cos
  Discrete-Time Integrator2 : DiscreteIntegrator  IntegratorMethod=Integration: Trapezoidal  SampleTime=-1  ICPrevOutput=DiscIntNeverNeededParam  ICPrevScaledInput=DiscIntNeverNeededParam
  Frq : Step  Time=FrqStpT  After=FrqStp*2*pi  SampleTime=0
  Gain : Gain  Gain=DcOff
  Harm : Step  Time=HarmStp  After=Harm  SampleTime=0  VectorParams1D=off
  Harm1 : Step  Time=IntHarmStp  After=IntHarm  SampleTime=0  VectorParams1D=off
  Mag : Step  Time=MagStpT  Before=1  After=MagStpPerc  SampleTime=0
  Matrix Multiply{,1..3} (4 alike) : Product  Multiplication=Matrix(*)
  Mod : Math  Operator=mod  SignedPower=on
  Phase : Step  Time=PhaStpT  After=(PhaStpPerc)*pi/180  SampleTime=0
  Product{,1,3,8} (4 alike) : Product
  Sum : Sum  Inputs=|++
  Sum of Elements : Sum  Inputs=+  CollapseMode=Specified dimension  CollapseDim=2
  Sum of Elements1 : Sum  Inputs=+  CollapseMode=Specified dimension  CollapseDim=2
  Sum of Elements2 : Sum  Inputs=+
  Sum1 : Sum  Inputs=|++
  Sum2 : Sum  Inputs=+--
  Sum3 : Sum  Inputs=++|
  Uact : Scope  NumInputPorts=2
  Wave : Outport  VectorParamsAs1DForOutWhenUnconnected=off
  wires:
  Sum of Elements2/1 -> Sum/2
  Mod/1 -> Uact/1  "wt_act"
  Constant5/1 -> Mod/2
  Gain/1 -> Sum3/1
  Sum3/1 -> Wave/1, Uact/2  "Uabc_act"
  Add7/1 -> Matrix Multiply/1, Matrix Multiply2/1, Cos3/1
  Product/1 -> Gain/1, Product3/2, Matrix Multiply1/1, Matrix Multiply3/1
  Matrix Multiply2/1 -> Cos1/1
  Matrix Multiply3/1 -> Product1/1
  Cos1/1 -> Product1/2
  Product1/1 -> Sum of Elements1/1
  Constant4/1 -> Matrix Multiply2/2
  Harm1/1 -> Matrix Multiply3/2
  Sum of Elements1/1 -> Sum2/3
  Sum2/1 -> Sum3/2
  Sum of Elements/1 -> Sum2/2
  Harm/1 -> Matrix Multiply1/2
  Constant3/1 -> Matrix Multiply/2
  Product8/1 -> Sum of Elements/1
  Cos8/1 -> Product8/2
  Matrix Multiply1/1 -> Product8/1
  Matrix Multiply/1 -> Cos8/1
  Constant2/1 -> Sum1/1
  Phase/1 -> Sum1/2
  Constant/1 -> Product/1
  Mag/1 -> Product/2
  Frq/1 -> Sum of Elements2/1
  Constant1/1 -> Sum/1
  Sum/1 -> Discrete-Time Integrator2/1
  Discrete-Time Integrator2/1 -> Add7/1, Mod/1  "wt_act"
  Product3/1 -> Sum2/1
  Sum1/1 -> Add7/2
  Cos3/1 -> Product3/1

== system GCI_Ctrl_PLL_C2000/PowerSystem/Meas/Fault Injection/TwoPhaseFault ==
  Add7 : Sum
  Constant : Constant  Value=Mag
  Constant1 : Constant  Value=Frq*2*pi
  Constant2 : Constant  Value=Pha*pi/180
  Constant3 : Constant  Value=HarmOrd  VectorParams1D=off
  Constant4 : Constant  Value=IntHarmOrd  VectorParams1D=off
  Constant5 : Constant  Value=2*pi
  Cos1 : Trigonometry  Operator=cos
  Cos3 : Trigonometry  Operator=cos
  Cos8 : Trigonometry  Operator=cos
  Dc : Step  Time=DcStpT  After=DcOff  SampleTime=0
  Discrete-Time Integrator2 : DiscreteIntegrator  IntegratorMethod=Integration: Trapezoidal  SampleTime=-1  ICPrevOutput=DiscIntNeverNeededParam  ICPrevScaledInput=DiscIntNeverNeededParam
  Frq : Step  Time=FrqStpT  After=FrqStp*2*pi  SampleTime=0
  Harm : Step  Time=HarmStp  After=Harm  SampleTime=0  VectorParams1D=off
  Harm1 : Step  Time=IntHarmStp  After=IntHarm  SampleTime=0  VectorParams1D=off
  Mag : Step  Time=MagStpT  Before=1  After=MagStpPerc  SampleTime=0
  Matrix Multiply{,1..3} (4 alike) : Product  Multiplication=Matrix(*)
  Mod : Math  Operator=mod  SignedPower=on
  Phase : Step  Time=PhaStpT  After=(PhaStpPerc)*pi/180  SampleTime=0
  Product{,1..3,8} (5 alike) : Product
  Sum : Sum  Inputs=|++
  Sum of Elements : Sum  Inputs=+  CollapseMode=Specified dimension  CollapseDim=2
  Sum of Elements1 : Sum  Inputs=+  CollapseMode=Specified dimension  CollapseDim=2
  Sum of Elements2 : Sum  Inputs=+
  Sum1 : Sum  Inputs=|++
  Sum2 : Sum  Inputs=+--
  Sum3 : Sum  Inputs=++|
  Uact : Scope  NumInputPorts=2
  Wave : Outport  VectorParamsAs1DForOutWhenUnconnected=off
  wires:
  Cos3/1 -> Product3/1
  Sum1/1 -> Add7/2
  Product3/1 -> Sum2/1
  Discrete-Time Integrator2/1 -> Mod/1, Add7/1  "wt_act"
  Sum/1 -> Discrete-Time Integrator2/1
  Constant1/1 -> Sum/1
  Frq/1 -> Sum of Elements2/1
  Mag/1 -> Product/2
  Constant/1 -> Product/1
  Phase/1 -> Sum1/2
  Constant2/1 -> Sum1/1
  Matrix Multiply/1 -> Cos8/1
  Matrix Multiply1/1 -> Product8/1
  Cos8/1 -> Product8/2
  Product8/1 -> Sum of Elements/1
  Constant3/1 -> Matrix Multiply/2
  Harm/1 -> Matrix Multiply1/2
  Sum of Elements/1 -> Sum2/2
  Sum2/1 -> Sum3/2
  Sum of Elements1/1 -> Sum2/3
  Harm1/1 -> Matrix Multiply3/2
  Constant4/1 -> Matrix Multiply2/2
  Product1/1 -> Sum of Elements1/1
  Cos1/1 -> Product1/2
  Matrix Multiply3/1 -> Product1/1
  Matrix Multiply2/1 -> Cos1/1
  Product/1 -> Product2/2, Matrix Multiply3/1, Matrix Multiply1/1, Product3/2
  Add7/1 -> Cos3/1, Matrix Multiply2/1, Matrix Multiply/1
  Sum3/1 -> Uact/2, Wave/1  "Uabc_act"
  Product2/1 -> Sum3/1
  Constant5/1 -> Mod/2
  Mod/1 -> Uact/1  "wt_act"
  Sum of Elements2/1 -> Sum/2
  Dc/1 -> Product2/1

== system GCI_Ctrl_PLL_C2000/PowerSystem/Plant/PWMGen1/Deadtime ==
  In1 : Inport
  AND : Logic  IconShape=distinctive  AllPortsSameDT=off  OutDataTypeStr=boolean
  Data Type Conversion : DataTypeConversion  OutDataTypeStr=double  SaturateOnIntegerOverflow=off  RndMeth=Floor
  Data Type Conversion1 : DataTypeConversion  SaturateOnIntegerOverflow=off  RndMeth=Floor
  Transport Delay : TransportDelay  DelayTime=double(Var.PWM.Freq)
  Out1 : Outport  VectorParamsAs1DForOutWhenUnconnected=off
  wires:
  Transport Delay/1 -> AND/1
  In1/1 -> Data Type Conversion/1
  AND/1 -> Data Type Conversion1/1
  Data Type Conversion/1 -> Transport Delay/1, AND/2
  Data Type Conversion1/1 -> Out1/1

== system GCI_Ctrl_PLL_C2000/PowerSystem/Plant/PWMGen2/Deadtime ==
  In1 : Inport
  AND : Logic  IconShape=distinctive  AllPortsSameDT=off  OutDataTypeStr=boolean
  Data Type Conversion : DataTypeConversion  OutDataTypeStr=double  SaturateOnIntegerOverflow=off  RndMeth=Floor
  Data Type Conversion1 : DataTypeConversion  SaturateOnIntegerOverflow=off  RndMeth=Floor
  Transport Delay : TransportDelay  DelayTime=double(Var.PWM.Freq)
  Out1 : Outport  VectorParamsAs1DForOutWhenUnconnected=off
  wires:
  Data Type Conversion1/1 -> Out1/1
  Data Type Conversion/1 -> AND/2, Transport Delay/1
  AND/1 -> Data Type Conversion1/1
  In1/1 -> Data Type Conversion/1
  Transport Delay/1 -> AND/1

== system GCI_Ctrl_PLL_C2000/C2000_SW/Control/CommunicationMode/Serial Receive/unParse ==
  Data : Inport
  Bitwise Operator : simulink/Logic and Bit Operations/Bitwise Operator  logicop=AND  UseBitMask=on  BitMask=1  BitMaskRealWorld=Stored Integer
  Bitwise Operator1 : simulink/Logic and Bit Operations/Bitwise Operator  logicop=AND  UseBitMask=on  BitMask=4  BitMaskRealWorld=Stored Integer
  Bitwise Operator2 : simulink/Logic and Bit Operations/Bitwise Operator  logicop=AND  UseBitMask=on  BitMask=2  BitMaskRealWorld=Stored Integer
  Bitwise Operator3 : simulink/Logic and Bit Operations/Bitwise Operator  logicop=AND  UseBitMask=on  BitMask=8  BitMaskRealWorld=Stored Integer
  Bitwise Operator4 : simulink/Logic and Bit Operations/Bitwise Operator  logicop=AND  UseBitMask=on  BitMask=16  BitMaskRealWorld=Stored Integer
  Bitwise Operator5 : simulink/Logic and Bit Operations/Bitwise Operator  logicop=AND  UseBitMask=on  BitMask=32  BitMaskRealWorld=Stored Integer
  Data Type Conversion{1..6} (6 alike) : DataTypeConversion  OutDataTypeStr=boolean  RndMeth=Simplest  SaturateOnIntegerOverflow=off
  Shift Arithmetic : ArithShift  BitShiftNumber=1
  Shift Arithmetic1 : ArithShift  BitShiftNumber=2
  Shift Arithmetic2 : ArithShift  BitShiftNumber=3
  Shift Arithmetic3 : ArithShift  BitShiftNumber=4
  Shift Arithmetic4 : ArithShift  BitShiftNumber=5
  ForcePwr : Outport
  TestTrigger : Outport  Port=2
  EnaMon : Outport  Port=3
  EnaPLL : Outport  Port=4
  P_or_I : Outport  Port=5
  Mod : Outport  Port=6
  wires:
  Bitwise Operator2/1 -> Shift Arithmetic/1
  Bitwise Operator1/1 -> Shift Arithmetic1/1
  Bitwise Operator/1 -> Data Type Conversion3/1
  Data Type Conversion1/1 -> EnaMon/1
  Shift Arithmetic1/1 -> Data Type Conversion1/1
  Data Type Conversion3/1 -> ForcePwr/1
  Shift Arithmetic/1 -> Data Type Conversion5/1
  Data Type Conversion5/1 -> TestTrigger/1
  Shift Arithmetic2/1 -> Data Type Conversion2/1
  Bitwise Operator3/1 -> Shift Arithmetic2/1
  Bitwise Operator4/1 -> Shift Arithmetic3/1
  Shift Arithmetic3/1 -> Data Type Conversion4/1
  Data Type Conversion4/1 -> P_or_I/1
  Data Type Conversion2/1 -> EnaPLL/1
  Shift Arithmetic4/1 -> Data Type Conversion6/1
  Bitwise Operator5/1 -> Shift Arithmetic4/1
  Data/1 -> Bitwise Operator/1, Bitwise Operator2/1, Bitwise Operator5/1, Bitwise Operator4/1, Bitwise Operator3/1, Bitwise Operator1/1
  Data Type Conversion6/1 -> Mod/1

== system GCI_Ctrl_PLL_C2000/C2000_SW/CtrlLoop/ADC Scaling/ADC Scaling 3 Cur/RemoveDCOffset ==
  VabcGrid : Inport
  Rst : Inport  Port=2
  LPF : Subsystem  VariantControl="Sim.FiltDcOff == \"LPF\""
  None : Subsystem  VariantControl="Sim.FiltDcOff == \"None\""
  VabcGridAdj : Outport  VectorParamsAs1DForOutWhenUnconnected=off
  VabcGridOff : Outport  Port=2  VectorParamsAs1DForOutWhenUnconnected=off

== system GCI_Ctrl_PLL_C2000/C2000_SW/CtrlLoop/ADC Scaling/ADC Scaling 3 Cur/Scaling ==
  CH : Inport
  Bias : Bias  Bias=-ADC_Off  SaturateOnIntegerOverflow=off
  Bias1 : Bias  Bias=-ADC_Off_Phy  SaturateOnIntegerOverflow=off
  Bus Creator : BusCreator  Inputs=2
  Data Type Conversion3 : DataTypeConversion  OutDataTypeStr=single  ConvertRealWorld=Stored Integer (SI)  SaturateOnIntegerOverflow=off  RndMeth=Floor
  Gain1 : Gain  Gain=ADC_Gain_Phy  OutDataTypeStr=single
  Gain2 : Gain  Gain=ADC_Gain  OutDataTypeStr=single
  Mon : Outport  Unit=V  VectorParamsAs1DForOutWhenUnconnected=off
  CH_Meas : Outport  Port=2  Unit=V  VectorParamsAs1DForOutWhenUnconnected=off
  wires:
  Gain1/1 -> CH_Meas/1, Bus Creator/2  "VaActMeas"
  Bias1/1 -> Gain1/1
  Bus Creator/1 -> Mon/1  "ScaleVaMon"
  Gain2/1 -> Bias1/1, Bus Creator/1  "VaPhyMeas"
  Bias/1 -> Gain2/1
  Data Type Conversion3/1 -> Bias/1
  CH/1 -> Data Type Conversion3/1

== system GCI_Ctrl_PLL_C2000/C2000_SW/CtrlLoop/ADC Scaling/ADC Scaling 3 Cur/Scaling1 ==
  CH : Inport
  Bias : Bias  Bias=-ADC_Off  SaturateOnIntegerOverflow=off
  Bias1 : Bias  Bias=-ADC_Off_Phy  SaturateOnIntegerOverflow=off
  Bus Creator : BusCreator  Inputs=2
  Data Type Conversion3 : DataTypeConversion  OutDataTypeStr=single  ConvertRealWorld=Stored Integer (SI)  SaturateOnIntegerOverflow=off  RndMeth=Floor
  Gain1 : Gain  Gain=ADC_Gain_Phy  OutDataTypeStr=single
  Gain2 : Gain  Gain=ADC_Gain  OutDataTypeStr=single
  Mon : Outport  Unit=V  VectorParamsAs1DForOutWhenUnconnected=off
  CH_Meas : Outport  Port=2  Unit=V  VectorParamsAs1DForOutWhenUnconnected=off
  wires:
  Gain1/1 -> CH_Meas/1, Bus Creator/2  "VbActMeas"
  Gain2/1 -> Bias1/1, Bus Creator/1  "VbPhyMeas"
  Bias1/1 -> Gain1/1
  Data Type Conversion3/1 -> Bias/1
  CH/1 -> Data Type Conversion3/1
  Bias/1 -> Gain2/1
  Bus Creator/1 -> Mon/1  "ScaleVbMon"

== system GCI_Ctrl_PLL_C2000/C2000_SW/CtrlLoop/ADC Scaling/ADC Scaling 3 Cur/Scaling2 ==
  CH : Inport
  Bias : Bias  Bias=-ADC_Off  SaturateOnIntegerOverflow=off
  Bias1 : Bias  Bias=-ADC_Off_Phy  SaturateOnIntegerOverflow=off
  Bus Creator : BusCreator  Inputs=2
  Data Type Conversion3 : DataTypeConversion  OutDataTypeStr=single  ConvertRealWorld=Stored Integer (SI)  SaturateOnIntegerOverflow=off  RndMeth=Floor
  Gain1 : Gain  Gain=ADC_Gain_Phy  OutDataTypeStr=single
  Gain2 : Gain  Gain=ADC_Gain  OutDataTypeStr=single
  Mon : Outport  VectorParamsAs1DForOutWhenUnconnected=off
  CH_Meas : Outport  Port=2  Unit=A  VectorParamsAs1DForOutWhenUnconnected=off
  wires:
  Bus Creator/1 -> Mon/1  "ScaleIaMon"
  Bias/1 -> Gain2/1
  Bias1/1 -> Gain1/1
  Data Type Conversion3/1 -> Bias/1
  CH/1 -> Data Type Conversion3/1
  Gain2/1 -> Bias1/1, Bus Creator/1  "IaPhyMeas"
  Gain1/1 -> CH_Meas/1, Bus Creator/2  "IaActMeas"

== system GCI_Ctrl_PLL_C2000/C2000_SW/CtrlLoop/ADC Scaling/ADC Scaling 3 Cur/Scaling3 ==
  CH : Inport
  Bias : Bias  Bias=-ADC_Off  SaturateOnIntegerOverflow=off
  Bias1 : Bias  Bias=-ADC_Off_Phy  SaturateOnIntegerOverflow=off
  Bus Creator : BusCreator  Inputs=2
  Data Type Conversion3 : DataTypeConversion  OutDataTypeStr=single  ConvertRealWorld=Stored Integer (SI)  SaturateOnIntegerOverflow=off  RndMeth=Floor
  Gain1 : Gain  Gain=ADC_Gain_Phy  OutDataTypeStr=single
  Gain2 : Gain  Gain=ADC_Gain  OutDataTypeStr=single
  Meas : Outport  VectorParamsAs1DForOutWhenUnconnected=off
  CH_Meas : Outport  Port=2  Unit=A  VectorParamsAs1DForOutWhenUnconnected=off
  wires:
  Bus Creator/1 -> Meas/1  "ScaleIbMon"
  Bias/1 -> Gain2/1
  Bias1/1 -> Gain1/1
  Data Type Conversion3/1 -> Bias/1
  CH/1 -> Data Type Conversion3/1
  Gain2/1 -> Bias1/1, Bus Creator/1  "IbPhyMeas"
  Gain1/1 -> CH_Meas/1, Bus Creator/2  "IbActMeas"

== system GCI_Ctrl_PLL_C2000/C2000_SW/CtrlLoop/ADC Scaling/ADC Scaling 3 Cur/Scaling4 ==
  CH : Inport
  Bias : Bias  Bias=-ADC_Off  SaturateOnIntegerOverflow=off
  Bias1 : Bias  Bias=-ADC_Off_Phy  SaturateOnIntegerOverflow=off
  Bus Creator : BusCreator  Inputs=2
  Data Type Conversion3 : DataTypeConversion  OutDataTypeStr=single  ConvertRealWorld=Stored Integer (SI)  SaturateOnIntegerOverflow=off  RndMeth=Floor
  Gain1 : Gain  Gain=ADC_Gain_Phy  OutDataTypeStr=single
  Gain2 : Gain  Gain=ADC_Gain  OutDataTypeStr=single
  Meas : Outport  VectorParamsAs1DForOutWhenUnconnected=off
  CH_Meas : Outport  Port=2  Unit=A  VectorParamsAs1DForOutWhenUnconnected=off
  wires:
  Bus Creator/1 -> Meas/1  "ScaleIcMon"
  Bias/1 -> Gain2/1
  Bias1/1 -> Gain1/1
  Data Type Conversion3/1 -> Bias/1
  CH/1 -> Data Type Conversion3/1
  Gain2/1 -> Bias1/1, Bus Creator/1  "IcPhyMeas"
  Gain1/1 -> CH_Meas/1, Bus Creator/2  "IcActMeas"

== system GCI_Ctrl_PLL_C2000/C2000_SW/CtrlLoop/ADC Scaling/ADC Scaling 3 Cur/Scaling5 ==
  CH : Inport
  Bias : Bias  Bias=-ADC_Off  SaturateOnIntegerOverflow=off
  Bias1 : Bias  Bias=-ADC_Off_Phy  SaturateOnIntegerOverflow=off
  Bus Creator : BusCreator  Inputs=2
  Data Type Conversion3 : DataTypeConversion  OutDataTypeStr=single  ConvertRealWorld=Stored Integer (SI)  SaturateOnIntegerOverflow=off  RndMeth=Floor
  Gain1 : Gain  Gain=ADC_Gain_Phy  OutDataTypeStr=single
  Gain2 : Gain  Gain=ADC_Gain  OutDataTypeStr=single
  Meas : Outport  Unit=V  VectorParamsAs1DForOutWhenUnconnected=off
  CH_Meas : Outport  Port=2  Unit=V  VectorParamsAs1DForOutWhenUnconnected=off
  wires:
  Bus Creator/1 -> Meas/1  "ScaleVdcMon"
  Bias/1 -> Gain2/1
  Bias1/1 -> Gain1/1
  Data Type Conversion3/1 -> Bias/1
  CH/1 -> Data Type Conversion3/1
  Gain2/1 -> Bias1/1, Bus Creator/1  "VdcPhyMeas"
  Gain1/1 -> CH_Meas/1, Bus Creator/2  "VdcActMeas"

== system GCI_Ctrl_PLL_C2000/C2000_SW/CtrlLoop/ADC Scaling/ADC Scaling 3 Cur/Subsystem ==
  IabcActMeas : Inport
  Enable : EnablePort
  LPF : Subsystem  mask{Ts=1/(Var.PWM_Freq), w=single(2*pi*5), K=single(1), y_0=0}
      mask prompts: Ts "Sample Time (s)"; w "CutOff Freq (-3db) (rad/s)"; K "Gain"; y_0 "Initial output"
  Saturation : Saturate  UpperLimit=5  LowerLimit=-5
  Offset : Outport
  wires:
  Saturation/1 -> Offset/1
  LPF/1(y) -> Saturation/1
  IabcActMeas/1 -> LPF/1(VabcGrid)

== system GCI_Ctrl_PLL_C2000/C2000_SW/CtrlLoop/ADC Scaling/ADC Scaling 3 Volts/RemoveDCOffset ==
  VabcGrid : Inport
  LPF : Subsystem  VariantControl="Sim.FiltDcOff == \"LPF\""
  None : Subsystem  VariantControl="Sim.FiltDcOff == \"None\""
  VabcGridAdj : Outport  VectorParamsAs1DForOutWhenUnconnected=off
  VabcGridOff : Outport  Port=2  VectorParamsAs1DForOutWhenUnconnected=off

== system GCI_Ctrl_PLL_C2000/C2000_SW/CtrlLoop/ADC Scaling/ADC Scaling 3 Volts/Scaling ==
  CH : Inport
  Bias : Bias  Bias=-ADC_Off  SaturateOnIntegerOverflow=off
  Bias1 : Bias  Bias=-ADC_Off_Phy  SaturateOnIntegerOverflow=off
  Bus Creator : BusCreator  Inputs=2
  Data Type Conversion3 : DataTypeConversion  OutDataTypeStr=single  ConvertRealWorld=Stored Integer (SI)  SaturateOnIntegerOverflow=off  RndMeth=Floor
  Gain1 : Gain  Gain=ADC_Gain_Phy  OutDataTypeStr=single
  Gain2 : Gain  Gain=ADC_Gain  OutDataTypeStr=single
  Mon : Outport  VectorParamsAs1DForOutWhenUnconnected=off
  CH_Meas : Outport  Port=2  VectorParamsAs1DForOutWhenUnconnected=off
  wires:
  CH/1 -> Data Type Conversion3/1
  Data Type Conversion3/1 -> Bias/1
  Bias/1 -> Gain2/1
  Gain2/1 -> Bus Creator/1, Bias1/1  "VaPhyMeas"
  Bus Creator/1 -> Mon/1  "ScaleVaMon"
  Bias1/1 -> Gain1/1
  Gain1/1 -> Bus Creator/2, CH_Meas/1  "VaActMeas"

== system GCI_Ctrl_PLL_C2000/C2000_SW/CtrlLoop/ADC Scaling/ADC Scaling 3 Volts/Scaling1 ==
  CH : Inport
  Bias : Bias  Bias=-ADC_Off  SaturateOnIntegerOverflow=off
  Bias1 : Bias  Bias=-ADC_Off_Phy  SaturateOnIntegerOverflow=off
  Bus Creator : BusCreator  Inputs=2
  Data Type Conversion3 : DataTypeConversion  OutDataTypeStr=single  ConvertRealWorld=Stored Integer (SI)  SaturateOnIntegerOverflow=off  RndMeth=Floor
  Gain1 : Gain  Gain=ADC_Gain_Phy  OutDataTypeStr=single
  Gain2 : Gain  Gain=ADC_Gain  OutDataTypeStr=single
  Mon : Outport  VectorParamsAs1DForOutWhenUnconnected=off
  CH_Meas : Outport  Port=2  VectorParamsAs1DForOutWhenUnconnected=off
  wires:
  Bus Creator/1 -> Mon/1  "ScaleVbMon"
  Bias/1 -> Gain2/1
  CH/1 -> Data Type Conversion3/1
  Data Type Conversion3/1 -> Bias/1
  Bias1/1 -> Gain1/1
  Gain2/1 -> Bus Creator/1, Bias1/1  "VbPhyMeas"
  Gain1/1 -> Bus Creator/2, CH_Meas/1  "VbActMeas"
